simulink model "simpleSignalParam"  (R2023b)
settings: Solver=VariableStepAuto  StartTime=0.0  StopTime=10.0  RelTol=1e-3
PreLoadFcn:
  | b = 3;
settings Model: Creator=grouleau  LastModifiedBy=grouleau

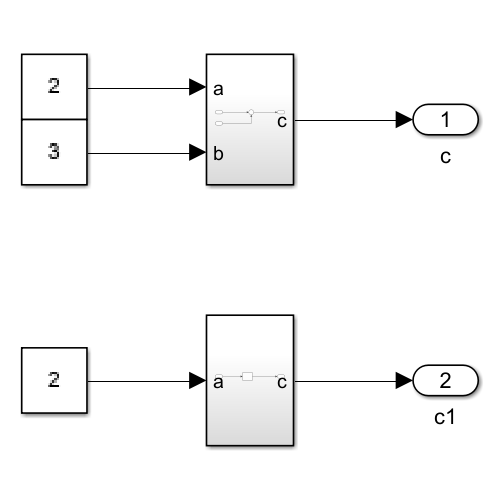
[thumbnail: Simulink's stored preview of the top-level diagram]
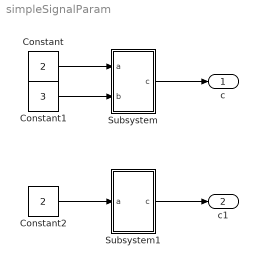
== system simpleSignalParam ==
  Constant : Constant  Value=2
  Constant1 : Constant  Value=3
  Constant2 : Constant  Value=2
  Subsystem : Subsystem
  Subsystem1 : Subsystem
  c : Outport
  c1 : Outport  Port=2
  wires:
  Constant/1 -> Subsystem/1(a)
  Constant1/1 -> Subsystem/2(b)
  Subsystem/1(c) -> c/1
  Subsystem1/1(c) -> c1/1
  Constant2/1 -> Subsystem1/1(a)

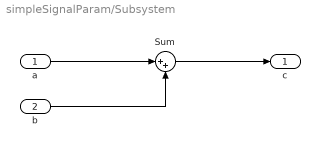
== system simpleSignalParam/Subsystem ==
  a : Inport
  b : Inport  Port=2
  Sum : Sum  Inputs=|++
  c : Outport
  wires:
  b/1 -> Sum/2
  a/1 -> Sum/1
  Sum/1 -> c/1

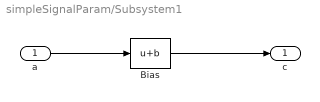
== system simpleSignalParam/Subsystem1 ==
  a : Inport
  Bias : Bias  Bias=b  SaturateOnIntegerOverflow=off
      settings: AttributesFormatString=b = 3
  c : Outport
  wires:
  Bias/1 -> c/1
  a/1 -> Bias/1
